simulink model "MS_BT_mdl_WS21"  (Simulink 9.2)
settings: Solver=FixedStepAuto  StartTime=0.0  StopTime=3  FixedStep=0.005  RelTol=1e-3
values from neighbouring files (symbols this model uses):
  cA = cE*(LE*cos(alp)/LR)^2    [MS_BT_mfile_WS21.m]
  cR = 128000    [MS_BT_mfile_WS21.m]
  cy = 70000    [MS_BT_mfile_WS21.m]
  cya = cy/ca    (= 3.5)    [MS_BT_mfile_WS21.m]
  dA = dE*(LE/LR)^2    (= 1150.2)    [MS_BT_mfile_WS21.m]
  ir = r/LR    (= 0.428571428571)    [MS_BT_mfile_WS21.m]
  mA = 229    [MS_BT_mfile_WS21.m]
  mR = 31    [MS_BT_mfile_WS21.m]
  v = 10    [MS_BT_mfile_WS21.m]
  Zh = 0.15    [MS_BT_mfile_WS21.m]
undefined symbols (not defined in the file or in its folder): sigbuilder_block
libraries: simulink x1
settings Model: Creator=wang  LastModifiedBy=wang
settings DataIOCC: LimitDataPoints=off  SaveFormat=Dataset  SignalLoggingSaveFormat=Dataset
settings OptimizationCC: LifeSpan=auto
settings DebuggingCC: UnderspecifiedInitializationDetection=Simplified  MergeDetectMultiDrivingBlocksExec=error  FcnCallInpInsideContextMsg=error  StateNameClashWarn=none  SFUnexpectedBacktrackingDiag=error  SFNoUnconditionalDefaultTransitionDiag=error  SFExecutionAtInitializationDiag=warning
settings HardwareCC: ProdBitPerPointer=64  ProdBitPerSizeT=64  ProdBitPerPtrDiffT=64  ProdLargestAtomicFloat=Float  ProdIntDivRoundTo=Zero  ProdEndianess=LittleEndian  ProdWordSize=64  ProdHWDeviceType=Intel->x86-64 (Windows64)
settings ModelReferenceCC: PropagateSignalLabelsOutOfModel=on
settings SFSimCC: SimUseLocalCustomCode=on
settings RTWCC: RTWUseLocalCustomCode=on
settings CodeAppCC: StateflowObjectComments=off
settings GRTTargetCC: TargetLangStandard=C99 (ISO)  GeneratePreprocessorConditionals=Use local settings  CombineOutputUpdateFcns=on  GRTInterface=off
settings ConfigComp: CovMetricSettings=dwe  CovHtmlReporting=off  CovSaveCumulativeToWorkspaceVar=off  CovSaveSingleToWorkspaceVar=off  CovExternalEMLEnable=on

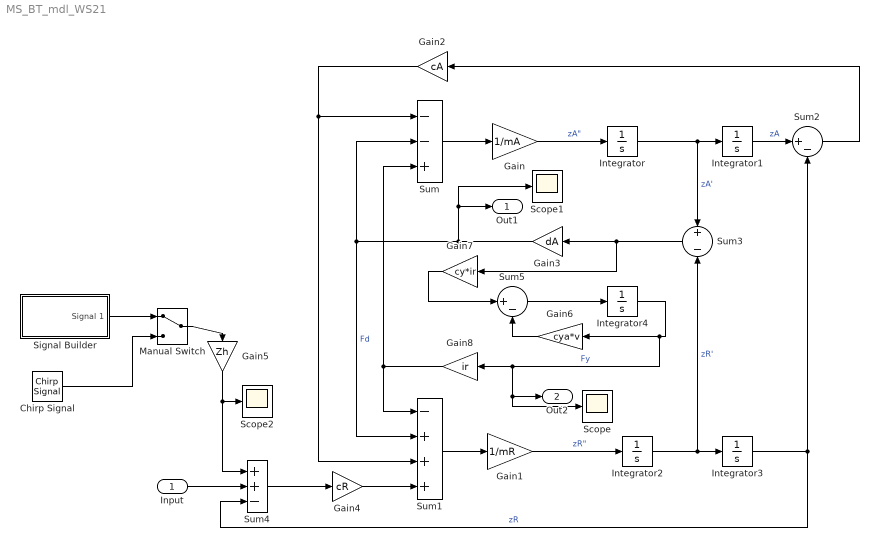
== system MS_BT_mdl_WS21 ==
  Input : Inport
  Chirp Signal : simulink/Sources/Chirp Signal  f1=0.01  T=20  f2=20
  Gain : Gain  Gain=1/mA
  Gain1 : Gain  Gain=1/mR
  Gain2 : Gain  Gain=cA
  Gain3 : Gain  Gain=dA
  Gain4 : Gain  Gain=cR
  Gain5 : Gain  Gain=Zh
  Gain6 : Gain  Gain=cya*v
  Gain7 : Gain  Gain=cy*ir
  Gain8 : Gain  Gain=ir
  Integrator{,1..4} (5 alike) : Integrator
  Manual Switch : ManualSwitch
  Scope : Scope
  Scope1 : Scope
  Scope2 : Scope
  Signal Builder : Subsystem  Tag=STV Subsys  LoadFcn=sigbuilder_block('load',[448.8 109.8 550.8 400.2 ]);  StartFcn=sigbuilder_block('start');  StopFcn=sigbuilder_block('stop');  ClipboardFcn=sigbuilder_block('clipboard');  mask(Sigbuilder block){tuvar=[0:10]}
      mask help: Simulink:masks:SigbuilderBlock_MD
      mask init:
      | if ~strcmp(get_param(bdroot(gcbh),'SimulationStatus'),'stopped') tuvar = sigbuilder_block('maskInit'); end
      settings: CopyFcn=sigbuilder_block('copy');  DeleteFcn=sigbuilder_block('delete');  ModelCloseFcn=sigbuilder_block('modelClose');  PreSaveFcn=sigbuilder_block('preSave');  PauseFcn=sigbuilder_block('pause');  ContinueFcn=sigbuilder_block('continue');  NameChangeFcn=sigbuilder_block('namechange');  OpenFcn=sigbuilder_block('open',[448.8 109.8 550.8 400.2 ]);  CloseFcn=sigbuilder_block('close');
      mask Display: plot(0, 0, 100, 100,[2, 2, 32, 32, 2], [68, 8, 8, 68, 68],[32, 2], [38, 38], [32, 19, 2],[53, 60, 44], [32, 17, 17, 2],[16, 16, 31, 31]);txt = getActiveGroup(gcbh);text(2, 100, txt,'verticalAlignment', 'top');
  Sum : Sum  Inputs=--+
  Sum1 : Sum  Inputs=-+++
  Sum2 : Sum  Inputs=|+-
  Sum3 : Sum  Inputs=+-
  Sum4 : Sum  Inputs=++-
  Sum5 : Sum  Inputs=|+-
  Out1 : Outport
  Out2 : Outport  Port=2
  wires:
  Sum/1 -> Gain/1
  Gain/1 -> Integrator/1  "zA\""
  Integrator/1 -> Sum3/1, Integrator1/1  "zA'"
  Integrator2/1 -> Integrator3/1, Sum3/2  "zR'"
  Sum1/1 -> Gain1/1
  Gain1/1 -> Integrator2/1  "zR\""
  Integrator1/1 -> Sum2/1  "zA"
  Integrator3/1 -> Sum2/2, Sum4/3  "zR"
  Sum2/1 -> Gain2/1
  Gain2/1 -> Sum1/3, Sum/1
  Sum3/1 -> Gain3/1, Gain7/1
  Gain4/1 -> Sum1/4
  Sum4/1 -> Gain4/1
  Gain5/1 -> Scope2/1, Sum4/1
  Signal Builder/1(Signal 1) -> Manual Switch/1
  Manual Switch/1 -> Gain5/1
  Chirp Signal/1 -> Manual Switch/2
  Input/1 -> Sum4/2
  Sum5/1 -> Integrator4/1
  Integrator4/1 -> Out2/1, Scope/1, Gain8/1, Gain6/1  "Fy"
  Gain6/1 -> Sum5/2
  Gain7/1 -> Sum5/1
  Gain8/1 -> Sum1/1, Sum/3
  Gain3/1 -> Scope1/1, Out1/1, Sum/2, Sum1/2  "Fd"

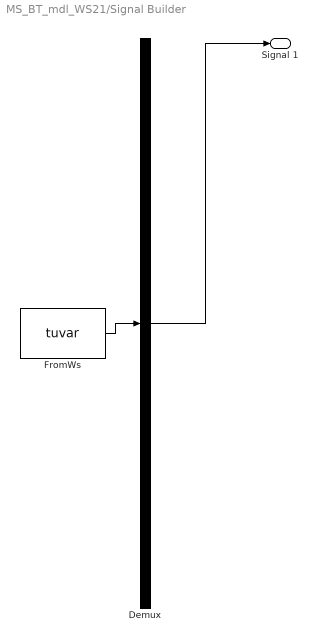
== system MS_BT_mdl_WS21/Signal Builder ==
  Demux : Demux  Tag=STV Demux  Outputs=1
  FromWs : FromWorkspace  Tag=STV FromWs  VariableName=tuvar  SampleTime=0  SigBuilderData=DataTag0  VnvData=DataTag1
      SigBuilderData=|
      | common.afterFinalStr = 'Extrapolate'
      | common.sampleTime = 0
      | dataSet.timeRange = [0 1]
      | dataSet.name = 'Group 1'
      | sbobj.Groups.Name = 'Group 1'
      | sbobj.Groups.Signals.Name = 'Signal 1'
      | sbobj.Groups.Signals.XData = [0 0.02 0.1 0.12 1]
      | sbobj.Groups.Signals.YData = [0 1 1 0 0]
      | sbobj.Groups.TimeRange = [0 1]
  Signal 1 : Outport  Tag=STV Outport
  wires:
  Demux/1 -> Signal 1/1
  FromWs/1 -> Demux/1
